simulink model "experiments"  (Simulink 8.0)
settings: Solver=ode45  StartTime=0.0  StopTime=10.0  RelTol=1e-3
settings Model: Creator=forrest  LastModifiedBy=forrest

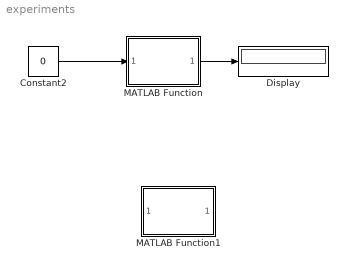
== system experiments ==
  Constant2 : Constant  Value=0
  Display : Display
  MATLAB Function : MATLAB Function  AncestorBlock=checkVoltage/checkVoltage/MATLAB Function  TreatAsAtomicUnit=on
  MATLAB Function1 : MATLAB Function  TreatAsAtomicUnit=on
  wires:
  Constant2/1 -> MATLAB Function/1(rmsVoltage)
  MATLAB Function/1(isWorking) -> Display/1

== matlab function MATLAB Function1 ==
  data: rmsVoltage input double; isWorking output double

function isWorking = checkRmsVoltage(rmsVoltage)

isWorking = 0;
if(rmsVoltage >= 110 && rmsVoltage <=120)
    isWorking = 1;

end

== matlab function MATLAB Function ==
  data: rmsVoltage input double; isWorking output double



function isWorking = checkRmsVoltage(rmsVoltage)

isWorking = 0;
if(rmsVoltage >= 110 && rmsVoltage <=120)
    isWorking = 1;

end
